simulink model "sampleModel1474"  (R2023a)
settings: Solver=VariableStepAuto  StartTime=0.0  StopTime=10.0  RelTol=1e-3
libraries: hdlsllib x2, simulink x1
settings Model: Creator=user1  LastModifiedBy=user1

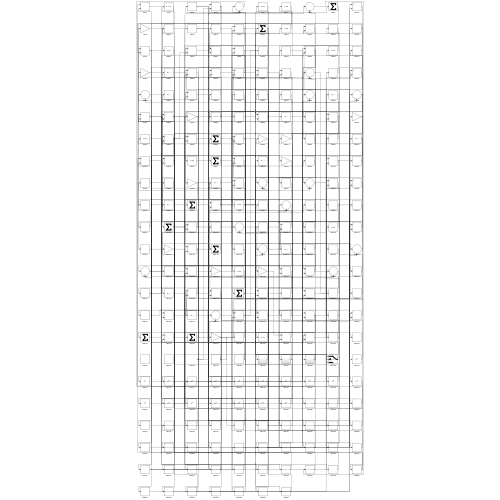
[thumbnail: Simulink's stored preview of the top-level diagram]
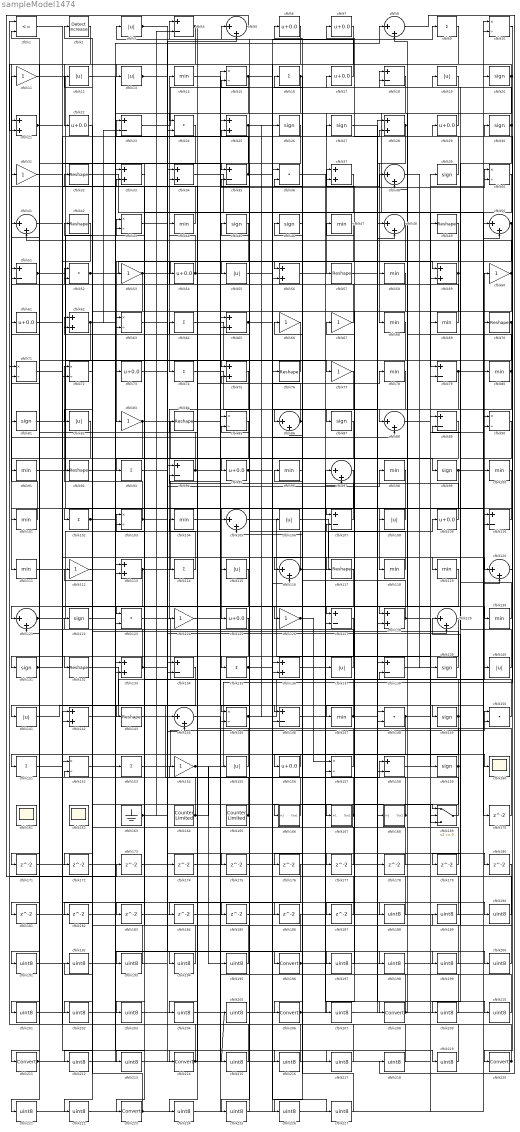
== system sampleModel1474 ==
  cfblk1 : RelationalOperator  Operator=<=  OutDataTypeStr=boolean  InputSameDT=off
  cfblk{10,15,40,43,63,71..72,85,90,103,145,152,157} (13 alike) : Product  Inputs=*/  RndMeth=Zero  SaturateOnIntegerOverflow=on
  cfblk{14,44,47,58,68..69,78,80,91,96,98,100..101,104,111,118..119,130,147} (19 alike) : MinMax
  cfblk{9,16,64,74,93,102,114,135,151,153} (10 alike) : Sum  Inputs=+
  cfblk{5,8,38,41,48,50,86,88,97,105,116,120..121,129,144} (15 alike) : Sum  Inputs=|++
  cfblk{3,12..13,19,55,82,106,108,115,137,140..141,155} (13 alike) : Abs  SaturateOnIntegerOverflow=off
  cfblk{4,18,23,35,51,79,89,94,107,110,127,134,138,146,158} (15 alike) : Sum  Inputs=+-
  cfblk{6..7,17,22,29,54,61,73,95,109,125,156} (12 alike) : Bias  Bias=0.0  SaturateOnIntegerOverflow=off
  cfblk{11,31,53,60,66..67,77,83,112,124,126,154} (12 alike) : Gain
  cfblk{21,25,28,33..34,37,56,59,62,65,75,113,128,133,136,142} (16 alike) : Sum
  cfblk{32,42,49,57,70,76,84,92,117,132,143} (11 alike) : Reshape
  cfblk{20,26..27,30,39,45..46,81,87,99,122,131,139,149,159} (15 alike) : Signum
  cfblk{24,36,52,123,148,150} (6 alike) : DotProduct  OutDataTypeStr=Inherit: Inherit via internal rule
  cfblk160 : Scope
  cfblk161 : Scope
      settings: Floating=on
  cfblk162 : Scope
      settings: Floating=on
  cfblk163 : Ground
  cfblk164 : hdlsllib/Sources/Counter Limited  uplimit=7  tsamp=-1
  cfblk165 : hdlsllib/Sources/Counter Limited  uplimit=7  tsamp=-1
  cfblk166 : Subsystem
      settings: LibrarySourceBlock=|
      | hdlsllib/Ports &
      | Subsystems/Subsystem
  cfblk167 : Subsystem
      settings: LibrarySourceBlock=|
      | hdlsllib/Ports &
      | Subsystems/Subsystem
  cfblk168 : Subsystem
      settings: LibrarySourceBlock=|
      | hdlsllib/Ports &
      | Subsystems/Subsystem
  cfblk169 : Switch  SaturateOnIntegerOverflow=off  InputSameDT=off
  cfblk{170..187} (18 alike) : Delay  SampleTime=1
  cfblk{188..195,197..205,207,209..210,212..213,215..219,221..222,224..227} (33 alike) : DataTypeConversion  OutDataTypeStr=uint8  SaturateOnIntegerOverflow=off  RndMeth=Floor
  cfblk{196,206,208,211,214,220,223} (7 alike) : DataTypeConversion  SaturateOnIntegerOverflow=off  RndMeth=Floor
  cfblk2 : simulink/Logic and Bit Operations/Detect Increase  vinit=0.0  OutDataTypeStr=boolean
      settings: LibrarySourceBlock=|
      | hdlsllib/Logic and Bit
      | Operations/Detect
      | Increase
  wires:
  cfblk38/1 -> cfblk139/1
  cfblk123/1 -> cfblk60/1
  cfblk108/1 -> cfblk102/1
  cfblk9/1 -> cfblk111/1
  cfblk101/1 -> cfblk11/1
  cfblk110/1 -> cfblk101/1
  cfblk154/1 -> cfblk29/1, cfblk195/1
  cfblk91/1 -> cfblk43/1
  cfblk105/1 -> cfblk159/1
  cfblk118/1 -> cfblk3/1
  cfblk48/1 -> cfblk74/1
  cfblk99/1 -> cfblk107/1, cfblk120/2
  cfblk11/1 -> cfblk125/1
  cfblk29/1 -> cfblk86/1
  cfblk46/1 -> cfblk116/1
  cfblk104/1 -> cfblk105/1
  cfblk135/1 -> cfblk5/1, cfblk169/1
  cfblk69/1 -> cfblk14/1
  cfblk54/1 -> cfblk44/1, cfblk146/1
  cfblk28/1 -> cfblk68/1, cfblk128/2
  cfblk75/1 -> cfblk124/1
  cfblk6/1 -> cfblk22/1
  cfblk51/1 -> cfblk77/1, cfblk186/1
  cfblk44/1 -> cfblk21/1
  cfblk151/1 -> cfblk142/1
  cfblk83/1 -> cfblk93/1, cfblk146/2
  cfblk126/1 -> cfblk16/1, cfblk157/1
  cfblk53/1 -> cfblk56/1, cfblk103/2
  cfblk22/1 -> cfblk132/1
  cfblk66/1 -> cfblk145/1
  cfblk168/1(Out1) -> cfblk167/1(In1), cfblk154/1
  cfblk87/1 -> cfblk121/1
  cfblk136/1 -> cfblk137/1
  cfblk18/1 -> cfblk57/1
  cfblk139/1 -> cfblk62/1
  cfblk147/1 -> cfblk43/2, cfblk48/2
  cfblk141/1 -> cfblk158/1
  cfblk159/1 -> cfblk67/1, cfblk202/1
  cfblk137/1 -> cfblk52/1
  cfblk169/1 -> cfblk45/1
  cfblk121/1 -> cfblk15/1, cfblk130/1
  cfblk158/1 -> cfblk49/1
  cfblk49/1 -> cfblk83/1
  cfblk156/1 -> cfblk151/1
  cfblk52/1 -> cfblk59/1, cfblk114/1
  cfblk78/1 -> cfblk88/1
  cfblk124/1 -> cfblk40/1
  cfblk92/1 -> cfblk126/1
  cfblk30/1 -> cfblk8/2, cfblk209/1
  cfblk79/1 -> cfblk136/2, cfblk80/1
  cfblk150/1 -> cfblk37/1
  cfblk17/1 -> cfblk4/1
  cfblk70/1 -> cfblk147/1, cfblk181/1
  cfblk56/1 -> cfblk119/1
  cfblk32/1 -> cfblk140/1
  cfblk102/1 -> cfblk8/1, cfblk219/1
  cfblk166/1(Out1) -> cfblk32/1
  cfblk133/1 -> cfblk61/1, cfblk98/1
  cfblk20/1 -> cfblk13/1, cfblk58/1
  cfblk12/1 -> cfblk99/1
  cfblk65/1 -> cfblk225/1, cfblk227/1
  cfblk163/1 -> cfblk34/1, cfblk4/2
  cfblk95/1 -> cfblk78/1, cfblk88/2, cfblk169/3
  cfblk10/1 -> cfblk220/1
  cfblk62/1 -> cfblk113/1, cfblk142/2, cfblk121/2, cfblk23/2
  cfblk167/1(Out1) -> cfblk41/1, cfblk187/1
  cfblk143/1 -> cfblk94/1
  cfblk134/1 -> cfblk211/1
  cfblk103/1 -> cfblk72/1, cfblk177/1
  cfblk149/1 -> cfblk35/2, cfblk176/1
  cfblk35/1 -> cfblk9/1, cfblk23/1
  cfblk16/1 -> cfblk63/2, cfblk86/2
  cfblk7/1 -> cfblk56/2
  cfblk42/1 -> cfblk72/2
  cfblk60/1 -> cfblk15/2, cfblk87/1, cfblk207/1
  cfblk74/1 -> cfblk138/1
  cfblk157/1 -> cfblk122/1
  cfblk47/1 -> cfblk196/1
  cfblk84/1 -> cfblk38/1
  cfblk14/1 -> cfblk115/1
  cfblk142/1 -> cfblk106/1
  cfblk131/1 -> cfblk37/2, cfblk28/2
  cfblk81/1 -> cfblk153/1
  cfblk34/1 -> cfblk79/1
  cfblk98/1 -> cfblk118/1
  cfblk113/1 -> cfblk65/1, cfblk123/1
  cfblk80/1 -> cfblk18/1, cfblk108/1
  cfblk146/1 -> cfblk149/1
  cfblk71/1 -> cfblk214/1
  cfblk153/1 -> cfblk150/1
  cfblk76/1 -> cfblk75/1
  cfblk109/1 -> cfblk94/2
  cfblk120/1 -> cfblk30/1
  cfblk37/1 -> cfblk156/1
  cfblk155/1 -> cfblk64/1
  cfblk88/1 -> cfblk79/2
  cfblk145/1 -> cfblk50/1, cfblk26/1
  cfblk115/1 -> cfblk143/1
  cfblk86/1 -> cfblk46/1, cfblk34/2
  cfblk4/1 -> cfblk21/2, cfblk24/1
  cfblk85/1 -> cfblk223/1
  cfblk114/1 -> cfblk104/1
  cfblk100/1 -> cfblk206/1
  cfblk129/1 -> cfblk166/1(In1)
  cfblk13/1 -> cfblk180/1, cfblk199/1
  cfblk132/1 -> cfblk168/1(In1)
  cfblk25/1 -> cfblk169/2, cfblk171/1
  cfblk31/1 -> cfblk35/1
  cfblk63/1 -> cfblk129/2
  cfblk138/1 -> cfblk90/2
  cfblk40/1 -> cfblk73/1
  cfblk107/1 -> cfblk66/1
  cfblk68/1 -> cfblk148/2
  cfblk82/1 -> cfblk131/1
  cfblk164/1 -> cfblk92/1, cfblk155/1
  cfblk50/1 -> cfblk95/1, cfblk65/2
  cfblk23/1 -> cfblk18/2
  cfblk165/1 -> cfblk103/1, cfblk51/1
  cfblk21/1 -> cfblk91/1, cfblk117/1
  cfblk55/1 -> cfblk17/1
  cfblk94/1 -> cfblk27/1, cfblk120/1, cfblk51/2
  cfblk39/1 -> cfblk7/1
  cfblk148/1 -> cfblk40/2, cfblk204/1, cfblk212/1
  cfblk111/1 -> cfblk53/1
  cfblk41/1 -> cfblk127/1
  cfblk117/1 -> cfblk141/1
  cfblk15/1 -> cfblk160/1, cfblk24/2
  cfblk67/1 -> cfblk31/1
  cfblk116/1 -> cfblk109/1, cfblk62/2
  cfblk128/1 -> cfblk150/2, cfblk105/2, cfblk81/1
  cfblk36/1 -> cfblk208/1
  cfblk59/1 -> cfblk82/1, cfblk128/1, cfblk41/2
  cfblk127/1 -> cfblk135/1
  cfblk64/1 -> cfblk116/2
  cfblk73/1 -> cfblk5/2
  cfblk140/1 -> cfblk19/1
  cfblk26/1 -> cfblk55/1
  cfblk130/1 -> cfblk89/2
  cfblk3/1 -> cfblk110/2, cfblk197/1
  cfblk77/1 -> cfblk127/2
  cfblk106/1 -> cfblk170/1
  cfblk170/1 -> cfblk107/2
  cfblk171/1 -> cfblk148/1
  cfblk89/1 -> cfblk172/1
  cfblk172/1 -> cfblk145/2
  cfblk5/1 -> cfblk173/1
  cfblk173/1 -> cfblk28/1
  cfblk43/1 -> cfblk174/1
  cfblk93/1 -> cfblk175/1
  cfblk175/1 -> cfblk59/2
  cfblk177/1 -> cfblk25/2
  cfblk57/1 -> cfblk178/1
  cfblk178/1 -> cfblk52/2
  cfblk90/1 -> cfblk179/1
  cfblk179/1 -> cfblk38/2
  cfblk181/1 -> cfblk133/2
  cfblk58/1 -> cfblk182/1
  cfblk182/1 -> cfblk113/2
  cfblk24/1 -> cfblk183/1
  cfblk183/1 -> cfblk136/1
  cfblk19/1 -> cfblk184/1
  cfblk184/1 -> cfblk50/2
  cfblk122/1 -> cfblk185/1
  cfblk187/1 -> cfblk6/1
  cfblk1/1 -> cfblk188/1
  cfblk188/1 -> cfblk12/1
  cfblk180/1 -> cfblk189/1
  cfblk189/1 -> cfblk1/1
  cfblk185/1 -> cfblk190/1
  cfblk190/1 -> cfblk1/2
  cfblk2/1 -> cfblk191/1
  cfblk191/1 -> cfblk54/1
  cfblk192/1 -> cfblk2/1
  cfblk33/1 -> cfblk193/1
  cfblk193/1 -> cfblk133/1
  cfblk45/1 -> cfblk194/1
  cfblk194/1 -> cfblk33/1
  cfblk195/1 -> cfblk33/2
  cfblk196/1 -> cfblk157/2, cfblk110/1
  cfblk197/1 -> cfblk47/1
  cfblk112/1 -> cfblk198/1
  cfblk198/1 -> cfblk70/1
  cfblk199/1 -> cfblk112/1
  cfblk144/1 -> cfblk200/1
  cfblk200/1 -> cfblk129/1
  cfblk125/1 -> cfblk201/1
  cfblk201/1 -> cfblk144/1
  cfblk202/1 -> cfblk144/2
  cfblk97/1 -> cfblk203/1
  cfblk203/1 -> cfblk90/1
  cfblk204/1 -> cfblk97/1
  cfblk205/1 -> cfblk97/2
  cfblk206/1 -> cfblk158/2, cfblk20/1, cfblk48/1
  cfblk207/1 -> cfblk100/1
  cfblk208/1 -> cfblk138/2, cfblk25/1
  cfblk209/1 -> cfblk36/1
  cfblk27/1 -> cfblk210/1
  cfblk210/1 -> cfblk36/2
  cfblk211/1 -> cfblk205/1, cfblk123/2, cfblk69/1
  cfblk212/1 -> cfblk134/1
  cfblk186/1 -> cfblk213/1
  cfblk213/1 -> cfblk134/2
  cfblk214/1 -> cfblk84/1, cfblk42/1
  cfblk174/1 -> cfblk215/1
  cfblk215/1 -> cfblk71/1
  cfblk61/1 -> cfblk216/1
  cfblk216/1 -> cfblk71/2
  cfblk152/1 -> cfblk217/1
  cfblk217/1 -> cfblk63/1
  cfblk8/1 -> cfblk218/1
  cfblk218/1 -> cfblk152/1
  cfblk219/1 -> cfblk152/2
  cfblk220/1 -> cfblk75/2, cfblk89/1
  cfblk119/1 -> cfblk221/1
  cfblk221/1 -> cfblk10/1
  cfblk72/1 -> cfblk222/1
  cfblk222/1 -> cfblk10/2
  cfblk223/1 -> cfblk192/1, cfblk76/1
  cfblk176/1 -> cfblk224/1
  cfblk224/1 -> cfblk85/1
  cfblk225/1 -> cfblk85/2
  cfblk96/1 -> cfblk226/1
  cfblk226/1 -> cfblk39/1
  cfblk227/1 -> cfblk96/1

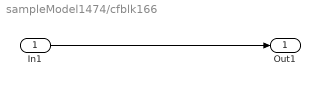
== system sampleModel1474/cfblk166 ==
  In1 : Inport
  Out1 : Outport
  wires:
  In1/1 -> Out1/1

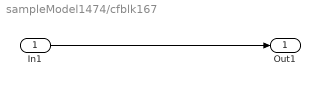
== system sampleModel1474/cfblk167 ==
  In1 : Inport
  Out1 : Outport
  wires:
  In1/1 -> Out1/1

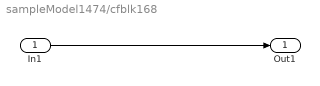
== system sampleModel1474/cfblk168 ==
  In1 : Inport
  Out1 : Outport
  wires:
  In1/1 -> Out1/1
